simulink model "hx_sim"  (R2017b)
settings: Solver=ode23tb  StartTime=0.0  StopTime=tEndSimul  MaxStep=0.1  RelTol=2.5e-6
values from neighbouring files (symbols this model uses):
  dnDt_in = mass_flow_converter(0, 'kg/min', 'mol/sec', 'Ammonia')    [hx.m]
  dnDt_out_liq = mass_flow_converter(0, 'kg/min', 'mol/sec', 'Ammonia')    [hx.m]
  dnDt_out_vap = mass_flow_converter(0.020, 'kg/min', 'mol/sec', 'Ammonia')    [hx.m]
  h_liq_wall = 1e4    (= 10000)    [hx.m]
  h_vap_wall = 1e2    (= 100)    [hx.m]
  h_wall_water = 200    [hx.m]
  L_min_water = 0.7    [hx.m]
  Shx_m2 = 0.351    [hx.m]
  T_dnDt_in_C = 0    [hx.m]
  tEnd_dnDt_in = tStart_dnDt_in + 0 * c.min_to_sec    [hx.m]
  tEnd_dnDt_out_liq = tStart_dnDt_out_liq + 0 * c.min_to_sec    [hx.m]
  tEnd_dnDt_out_vap = tStart_dnDt_out_vap + 10 * c.min_to_sec    [hx.m]
  tEndSimul = tEnd_dnDt_out_vap + 5 * c.min_to_sec    [hx.m]
  tStart_dnDt_in = 0 * c.min_to_sec    [hx.m]
  tStart_dnDt_out_liq = 0 * c.min_to_sec    [hx.m]
  tStart_dnDt_out_vap = 20 * c.min_to_sec    [hx.m]
  Twater_in_C = 10    [hx.m]
undefined symbols (not defined in the file or in its folder): h, P, T
libraries: thermochemical x9, simulink x1
settings Model: Creator=ferru  LastModifiedBy=fferrucc
settings SolverCC: AlgebraicLoopSolver=LineSearch

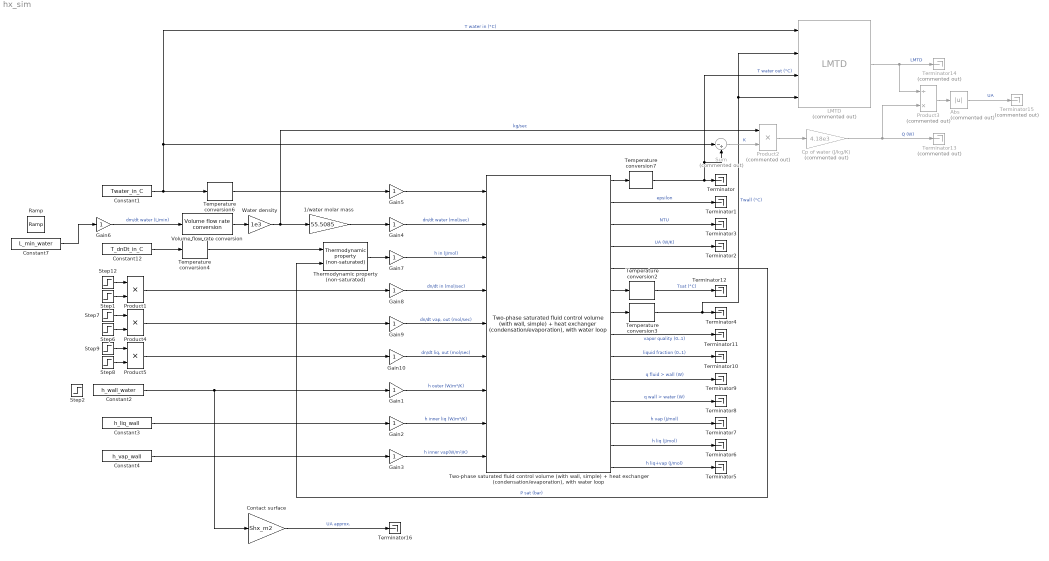
== system hx_sim ==
  1/water molar mass : Gain  Gain=55.5085
  Abs : Abs  Commented=on  ZeroCross=off
  Constant1 : Constant  Value=Twater_in_C
  Constant12 : Constant  Value=T_dnDt_in_C
  Constant2 : Constant  Value=h_wall_water
  Constant3 : Constant  Value=h_liq_wall
  Constant4 : Constant  Value=h_vap_wall
  Constant7 : Constant  Value=L_min_water
  Contact surface : Gain  Gain=Shx_m2
  Cp of water (J/kg/K) : Gain  Commented=on  Gain=4.18e3
  Gain{1..10} (10 alike) : Gain
  LMTD : thermochemical/Heat exchangers/LMTD  Commented=on
      settings: SourceProductName=@ Thermochemical
  Product1 : Product
  Product2 : Product  Commented=on
  Product3 : Product  Commented=on  Inputs=/*
  Product4 : Product
  Product5 : Product
  Ramp : simulink/Sources/Ramp  slope=2*L_min_water/tEndSimul  start=0  X0=L_min_water
  Step1 : Step  Time=tEnd_dnDt_in  Before=1  After=0  SampleTime=0
  Step12 : Step  Time=tStart_dnDt_in  After=dnDt_in  SampleTime=0
  Step2 : Step  Time=100  Before=200  After=400  SampleTime=0  ZeroCross=off
  Step6 : Step  Time=tEnd_dnDt_out_vap  Before=1  After=0  SampleTime=0
  Step7 : Step  Time=tStart_dnDt_out_vap  After=dnDt_out_vap  SampleTime=0
  Step8 : Step  Time=tEnd_dnDt_out_liq  Before=1  After=0  SampleTime=0
  Step9 : Step  Time=tStart_dnDt_out_liq  After=dnDt_out_liq  SampleTime=0
  Sum : Sum  Commented=on  Inputs=|-+
  Temperature conversion2 : thermochemical/Conversions/Temperature conversion  sel=K --> °C
      settings: SourceProductName=@ Thermochemical
  Temperature conversion3 : thermochemical/Conversions/Temperature conversion  sel=K --> °C
      settings: SourceProductName=@ Thermochemical
  Temperature conversion4 : thermochemical/Conversions/Temperature conversion  sel=°C --> K
      settings: SourceProductName=@ Thermochemical
  Temperature conversion6 : thermochemical/Conversions/Temperature conversion  sel=°C --> K
      settings: SourceProductName=@ Thermochemical
  Temperature conversion7 : thermochemical/Conversions/Temperature conversion  sel=K --> °C
      settings: SourceProductName=@ Thermochemical
  Terminator{,1..12,16} (14 alike) : Terminator
  Terminator13 : Terminator  Commented=on
  Terminator14 : Terminator  Commented=on
  Terminator15 : Terminator  Commented=on
  Thermodynamic property (non-saturated) : thermochemical/Thermodynamic fluid properties/Thermodynamic  property (non-saturated)  sel=h(T,P)  fluid=fluid  reciprocVar=-1  lookup2D_BreakPoint1=fluid.no_sat.T_P_indep.var_indep.T  lookup2D_BreakPoint2=fluid.no_sat.T_P_indep.var_indep.P  lookup2D_Data=fluid.no_sat.T_P_indep.var_dep.h_molar
      settings: SourceProductName=@ Thermochemical
  "Two-phase saturated fluid control volume (with wall, simple) + heat exchanger (condensation/evaporation), with water loop" : thermochemical/Control volumes/Two-phase saturated fluid control volume (with wall, simple) + heat exchanger (condensation//evaporation), with water loop
      link override "Two-phase saturated fluid control volume (with wall, simple)/Two-phase saturated fluid control volume (without walls)": N_init=Nhx_init  T_init=Thx_init  V=Vhx
      link override "Two-phase saturated fluid control volume (with wall, simple)/Wall, simple, h as inputs": material=Stainless steel AISI316  cp=490.8  rho=8023  s=Shx_m2  e_mm=thickness_hx_mm  mass=2.2529
      settings: SourceProductName=@ Thermochemical
  Volume flow rate conversion : thermochemical/Conversions/Volume flow rate conversion  sel=L/min --> m3/sec
      settings: SourceProductName=@ Thermochemical
  Water density : Gain  Gain=1e3
  wires:
  Step12/1 -> Product1/1
  Step1/1 -> Product1/2
  Constant12/1 -> Temperature conversion4/1
  Temperature conversion4/1 -> Thermodynamic property (non-saturated)/1
  Temperature conversion2/1 -> Terminator12/1  "Tsat (°C)"
  "Two-phase saturated fluid control volume (with wall, simple) + heat exchanger (condensation/evaporation), with water loop"/6 -> Temperature conversion2/1
  Gain7/1 -> "Two-phase saturated fluid control volume (with wall, simple) + heat exchanger (condensation/evaporation), with water loop"/3  "h in (J/mol)"
  Gain8/1 -> "Two-phase saturated fluid control volume (with wall, simple) + heat exchanger (condensation/evaporation), with water loop"/4  "dn/dt in (mol/sec)"
  Gain9/1 -> "Two-phase saturated fluid control volume (with wall, simple) + heat exchanger (condensation/evaporation), with water loop"/5  "dn/dt vap, out (mol/sec)"
  Gain10/1 -> "Two-phase saturated fluid control volume (with wall, simple) + heat exchanger (condensation/evaporation), with water loop"/6  "dn/dt liq, out (mol/sec)"
  "Two-phase saturated fluid control volume (with wall, simple) + heat exchanger (condensation/evaporation), with water loop"/5 -> Thermodynamic property (non-saturated)/2  "P sat (bar)"
  "Two-phase saturated fluid control volume (with wall, simple) + heat exchanger (condensation/evaporation), with water loop"/9 -> Terminator10/1  "liquid fraction (0..1)"
  "Two-phase saturated fluid control volume (with wall, simple) + heat exchanger (condensation/evaporation), with water loop"/8 -> Terminator11/1  "vapor quality (0..1)"
  "Two-phase saturated fluid control volume (with wall, simple) + heat exchanger (condensation/evaporation), with water loop"/12 -> Terminator7/1  "h vap (J/mol)"
  "Two-phase saturated fluid control volume (with wall, simple) + heat exchanger (condensation/evaporation), with water loop"/14 -> Terminator5/1  "h liq+vap (J/mol)"
  "Two-phase saturated fluid control volume (with wall, simple) + heat exchanger (condensation/evaporation), with water loop"/13 -> Terminator6/1  "h liq (J/mol)"
  Constant1/1 -> LMTD/1, Sum/1, Temperature conversion6/1  "T water in (°C)"
  Thermodynamic property (non-saturated)/1 -> Gain7/1
  Product1/1 -> Gain8/1
  Product4/1 -> Gain9/1
  Step6/1 -> Product4/2
  Step7/1 -> Product4/1
  Step9/1 -> Product5/1
  Step8/1 -> Product5/2
  Product5/1 -> Gain10/1
  "Two-phase saturated fluid control volume (with wall, simple) + heat exchanger (condensation/evaporation), with water loop"/7 -> Temperature conversion3/1
  Temperature conversion3/1 -> LMTD/4, LMTD/2, Terminator4/1  "Twall (°C)"
  "Two-phase saturated fluid control volume (with wall, simple) + heat exchanger (condensation/evaporation), with water loop"/11 -> Terminator8/1  "q wall > water (W)"
  "Two-phase saturated fluid control volume (with wall, simple) + heat exchanger (condensation/evaporation), with water loop"/10 -> Terminator9/1  "q fluid > wall (W)"
  Temperature conversion7/1 -> LMTD/3, Sum/2, Terminator/1  "T water out (°C)"
  Gain3/1 -> "Two-phase saturated fluid control volume (with wall, simple) + heat exchanger (condensation/evaporation), with water loop"/9  "h inner vap(W/m²/K)"
  Gain1/1 -> "Two-phase saturated fluid control volume (with wall, simple) + heat exchanger (condensation/evaporation), with water loop"/7  "h outer (W/m²/K)"
  Gain2/1 -> "Two-phase saturated fluid control volume (with wall, simple) + heat exchanger (condensation/evaporation), with water loop"/8  "h inner liq (W/m²/K)"
  Constant2/1 -> Contact surface/1, Gain1/1
  Constant3/1 -> Gain2/1
  Constant4/1 -> Gain3/1
  Temperature conversion6/1 -> Gain5/1
  Volume flow rate conversion/1 -> Water density/1
  1/water molar mass/1 -> Gain4/1
  Water density/1 -> Product2/1, 1/water molar mass/1  "kg/sec"
  "Two-phase saturated fluid control volume (with wall, simple) + heat exchanger (condensation/evaporation), with water loop"/4 -> Terminator2/1  "UA (W/K)"
  "Two-phase saturated fluid control volume (with wall, simple) + heat exchanger (condensation/evaporation), with water loop"/3 -> Terminator3/1  "NTU"
  "Two-phase saturated fluid control volume (with wall, simple) + heat exchanger (condensation/evaporation), with water loop"/1 -> Temperature conversion7/1
  "Two-phase saturated fluid control volume (with wall, simple) + heat exchanger (condensation/evaporation), with water loop"/2 -> Terminator1/1  "epsilon"
  Gain4/1 -> "Two-phase saturated fluid control volume (with wall, simple) + heat exchanger (condensation/evaporation), with water loop"/2  "dn/dt water (mol/sec)"
  Gain5/1 -> "Two-phase saturated fluid control volume (with wall, simple) + heat exchanger (condensation/evaporation), with water loop"/1
  Sum/1 -> Product2/2  "K"
  Product2/1 -> Cp of water (J/kg/K)/1
  Cp of water (J/kg/K)/1 -> Terminator13/1, Product3/2  "Q (W)"
  LMTD/1 -> Product3/1, Terminator14/1  "LMTD"
  Product3/1 -> Abs/1
  Abs/1 -> Terminator15/1  "UA"
  Contact surface/1 -> Terminator16/1  "UA approx."
  Gain6/1 -> Volume flow rate conversion/1  "dm/dt water (L/min)"
  Constant7/1 -> Gain6/1
